simulink model "Set_ACC_DEC_Spee_BSP"  (R2015a)
settings: Solver=FixedStepDiscrete  SolverMode=SingleTasking  StartTime=0.0  StopTime=10.0  FixedStep=1e-3  RelTol=1e-3
libraries: mbed_spi_power x9, mbed_lib x4
settings Model: Creator=svenl  LastModifiedBy=svenl
settings OptimizationCC: OptimizeModelRefInitCode=on  LifeSpan=1
settings HardwareCC: ProdLargestAtomicInteger=Long  ProdLargestAtomicFloat=Double  ProdEndianess=LittleEndian  ProdHWDeviceType=ARM Compatible->ARM Cortex
settings RTWCC: SystemTargetFile=mbed.tlc  TemplateMakefile=mbed.tmf  Description=Mbed Target (Embedded Target)  TargetLang=C++
settings CodeAppCC: IgnoreCustomStorageClasses=off
settings STFCustomTargetCC: CombineOutputUpdateFcns=on  SupportContinuousTime=off  SupportVariableSizeSignals=off  SystemTargetFile=mbed.tlc
settings ERTTargetCC: SupportContinuousTime=off  SupportVariableSizeSignals=off  ERTCustomFileTemplate=mbed_file_process.tlc

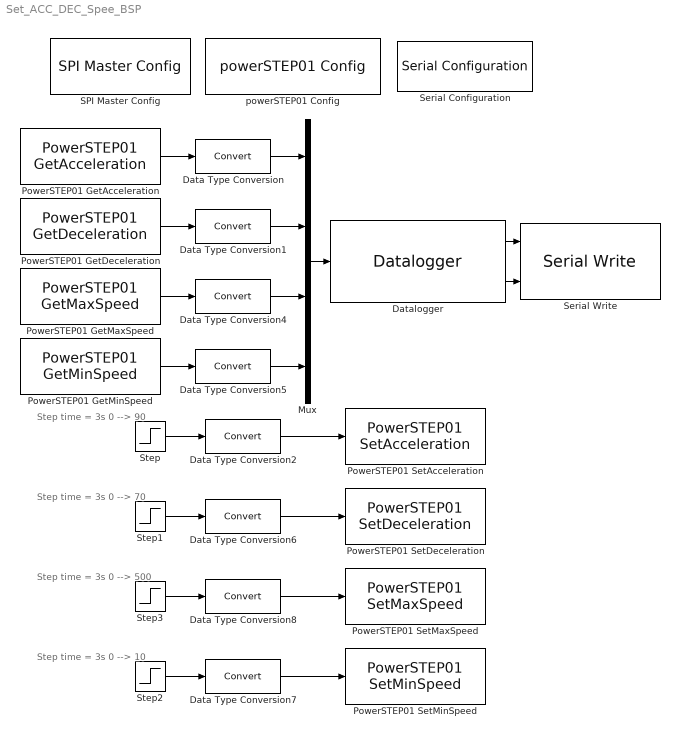
== system Set_ACC_DEC_Spee_BSP ==
  note: Step time = 3s
      | 0 --> 90
  note: Step time = 3s
      | 0 --> 70
  note: Step time = 3s
      | 0 --> 10
  note: Step time = 3s
      | 0 --> 500
  Data Type Conversion{,1..2,4..8} (8 alike) : DataTypeConversion
  Datalogger : mbed_lib/Utilities/Datalogger  TypeInputPorts={ 'double' 4 }  TypeOfInputs={'4*double'}  BufferSize=10000  errEn=off  SampleTime=-1
  Mux : Mux
  PowerSTEP01 GetAcceleration : mbed_spi_power/PowerSTEP01 GetAcceleration  SPINr=1  NumMotors=1  SSELPort=B  SSELPin=6  SampleTime=-1
  PowerSTEP01 GetDeceleration : mbed_spi_power/PowerSTEP01 GetDeceleration  SPINr=1  NumMotors=1  SSELPort=B  SSELPin=6  SampleTime=-1
  PowerSTEP01 GetMaxSpeed : mbed_spi_power/PowerSTEP01 GetMaxSpeed  SPINr=1  NumMotors=1  SSELPort=B  SSELPin=6  SampleTime=-1
  PowerSTEP01 GetMinSpeed : mbed_spi_power/PowerSTEP01 GetMinSpeed  SPINr=1  NumMotors=1  SSELPort=B  SSELPin=6  SampleTime=-1
  PowerSTEP01 SetAcceleration : mbed_spi_power/PowerSTEP01 SetAcceleration  SPINr=1  NumMotors=1  SSELPort=B  SSELPin=6  SampleTime=-1
  PowerSTEP01 SetDeceleration : mbed_spi_power/PowerSTEP01 SetDeceleration  SPINr=1  NumMotors=1  SSELPort=B  SSELPin=6  SampleTime=-1
  PowerSTEP01 SetMaxSpeed : mbed_spi_power/PowerSTEP01 SetMaxSpeed  SPINr=1  NumMotors=1  SSELPort=B  SSELPin=6  SampleTime=-1
  PowerSTEP01 SetMinSpeed : mbed_spi_power/PowerSTEP01 SetMinSpeed  SPINr=1  NumMotors=1  SSELPort=B  SSELPin=6  SampleTime=-1
  SPI Master Config : mbed_lib/SPI/SPI Master Config  Priority=0  SpiPort=1  SpiFreq=100000  MosiPort=A  MosiPin=7  MisoPort=A  MisoPin=6  SclkPort=A  SclkPin=5
  Serial Configuration : mbed_lib/Serial/Serial Configuration  SerialPort=1  TXPort=A  TXPin=2  RXPort=A  RXPin=3  BaudRate=115200
  Serial Write : mbed_lib/Serial/Serial Write  SerialPort=1  numData=on  SampleTime=0.01
  Step : Step  Time=3  After=90  SampleTime=0.1
  Step1 : Step  Time=3  After=70  SampleTime=0.1
  Step2 : Step  Time=3  After=10  SampleTime=0.1
  Step3 : Step  Time=3  After=500  SampleTime=0.1
  powerSTEP01 Config : mbed_spi_power/powerSTEP01 Config  Priority=0  SPINr=1  SSELPort=B  SSELPin=6  ResetPort=A  ResetPin=9  ACC=50  DEC=50  MaxSpeed=200  MinSpeed=0  FullStepSpeed=150  Overcurrent=100  StepMode=STEP_MODE_1_128  Holdtorque=20  Runtorque=20  ACCtorque=20  DECtorque=20  Motor2SEL=on  ACC_1=50  DEC_1=50  MaxSpeed_1=500  MinSpeed_1=0  FullStepSpeed_1=350  Overcurrent_1=150  StepMode_1=STEP_MODE_1_32  Holdtorque_1=50  Runtorque_1=50  ACCtorque_1=50  DECtorque_1=50  Motor3SEL=off  ACC_2=0  DEC_2=0  MaxSpeed_2=0  MinSpeed_2=0  FullStepSpeed_2=0  Overcurrent_2=0  StepMode_2=STEP_MODE_FULL  Holdtorque_2=0  Runtorque_2=0  ACCtorque_2=0  DECtorque_2=0
  wires:
  Datalogger/1 -> Serial Write/1
  Datalogger/2 -> Serial Write/2
  Mux/1 -> Datalogger/1
  Step/1 -> Data Type Conversion2/1
  Data Type Conversion2/1 -> PowerSTEP01 SetAcceleration/1
  PowerSTEP01 GetMinSpeed/1 -> Data Type Conversion5/1
  PowerSTEP01 GetMaxSpeed/1 -> Data Type Conversion4/1
  PowerSTEP01 GetDeceleration/1 -> Data Type Conversion1/1
  PowerSTEP01 GetAcceleration/1 -> Data Type Conversion/1
  Data Type Conversion5/1 -> Mux/4
  Step1/1 -> Data Type Conversion6/1
  Data Type Conversion6/1 -> PowerSTEP01 SetDeceleration/1
  Data Type Conversion7/1 -> PowerSTEP01 SetMinSpeed/1
  Data Type Conversion8/1 -> PowerSTEP01 SetMaxSpeed/1
  Step3/1 -> Data Type Conversion8/1
  Step2/1 -> Data Type Conversion7/1
  Data Type Conversion/1 -> Mux/1
  Data Type Conversion1/1 -> Mux/2
  Data Type Conversion4/1 -> Mux/3
